simulink model "IntegratedpmsmmotorofEV"  (R2025b)
settings: Solver=VariableStepAuto  StartTime=0.0  StopTime=400  RelTol=1e-3
values from neighbouring files (symbols this model uses):
  av = 1 / 1.475    (= 0.677966101695)    [variable_initialization.m]
  ig = 9    [variable_initialization.m]
  Ld = 1e-4    (= 0.0001)    [variable_initialization.m]
  phi = 0.23    [variable_initialization.m]
  Reff = 0.3    [variable_initialization.m]
  Rs = 0.00475    [variable_initialization.m]
  Zp = 3    [variable_initialization.m]
libraries: slpidlib x2
settings Model: Creator=HS TRADER  LastModifiedBy=sheik
settings RTWCC: GPUComputeCapability=3.5

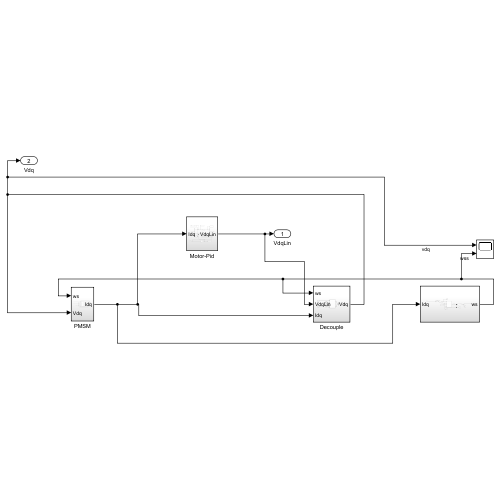
[thumbnail: Simulink's stored preview of the top-level diagram]
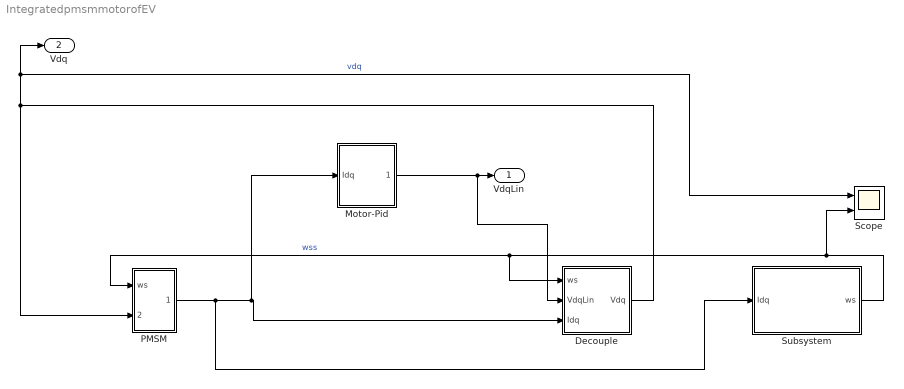
== system IntegratedpmsmmotorofEV ==
  Decouple : Subsystem
  Motor-Pid : Subsystem
  PMSM : Subsystem
  Scope : Scope  NumInputPorts=2
      settings: ActiveDisplayYMinimum=-1  ActiveDisplayYMaximum=1  DataLoggingVariableName=ScopeData2
  Subsystem : Subsystem
  VdqLin : Outport
  Vdq : Outport  Port=2
  wires:
  Motor-Pid/1(VdqLin) -> Decouple/2(VdqLin), VdqLin/1
  Decouple/1(Vdq) -> PMSM/2(Vdq), Scope/1, Vdq/1  "vdq"
  PMSM/1(Idq) -> Subsystem/1(Idq), Motor-Pid/1(Idq), Decouple/3(Idq)
  Subsystem/1(ws) -> Scope/2, Decouple/1(ws), PMSM/1(ws)  "wss"

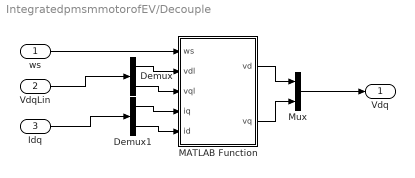
== system IntegratedpmsmmotorofEV/Decouple ==
  ws : Inport
  VdqLin : Inport  Port=2
  Idq : Inport  Port=3
  Demux : Demux  Outputs=2
  Demux1 : Demux  Outputs=2
  MATLAB Function : MATLAB Function  TreatAsAtomicUnit=on
  Mux : Mux  Inputs=2
  Vdq : Outport
  wires:
  Demux1/2 -> MATLAB Function/5(id)
  Demux/2 -> MATLAB Function/3(vql)
  Mux/1 -> Vdq/1
  Demux/1 -> MATLAB Function/2(vdl)
  MATLAB Function/1(vd) -> Mux/1
  VdqLin/1 -> Demux/1
  ws/1 -> MATLAB Function/1(ws)
  Demux1/1 -> MATLAB Function/4(iq)
  MATLAB Function/2(vq) -> Mux/2
  Idq/1 -> Demux1/1

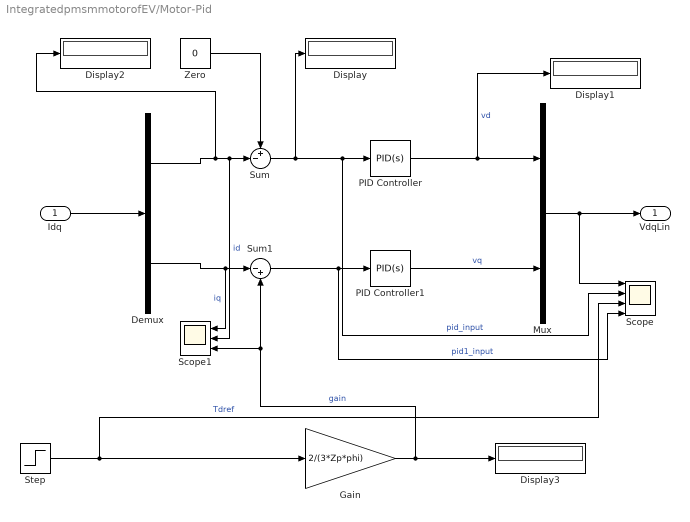
== system IntegratedpmsmmotorofEV/Motor-Pid ==
  Idq : Inport
  Demux : Demux  Outputs=2
  Display{,1..3} (4 alike) : Display
  Gain : Gain  Gain=2/(3*Zp*phi)
  Mux : Mux  Inputs=2
  PID Controller : slpidlib/PID Controller  Controller=PID  Form=Parallel  TimeDomain=Continuous-time  UseExternalTs=off  SampleTime=-1  IntegratorMethod=Forward Euler  FilterMethod=Forward Euler  ControllerParametersSource=internal  P=av  I=(Rs/Ld)*av  UseKiTs=off  D=0  UseExternalDerivativeSource=off  N=100  UseFilter=on  TunerSelectOption=Transfer Function Based (PID Tuner App)  InitialConditionSource=internal  InitialConditionForIntegrator=0  InitialConditionForFilter=0  DifferentiatorICPrevScaledInput=0  ExternalReset=none  TrackingMode=off  Kt=1  LimitOutput=off  SatLimitsSource=internal  UpperSaturationLimit=inf  LowerSaturationLimit=-inf  LinearizeAsGain=on  AntiWindupMode=none  Kb=1  LimitIntegrator=off  UpperIntegratorSaturationLimit=inf  LowerIntegratorSaturationLimit=-inf  POutMin=[]  POutMax=[]  IOutMin=[]  IOutMax=[]  DOutMin=[]  DOutMax=[]  NOutMin=[]  NOutMax=[]  SumOutMin=[]  SumOutMax=[]  SaturationOutMin=[]  SaturationOutMax=[]  PParamMin=[]  PParamMax=[]  IParamMin=[]  IParamMax=[]  DParamMin=[]  DParamMax=[]  NParamMin=[]  NParamMax=[]  KbParamMin=[]  KbParamMax=[]  KtParamMin=[]  KtParamMax=[]  KbOutMin=[]  KbOutMax=[]  KtOutMin=[]  KtOutMax=[]  IntegratorOutMin=[]  IntegratorOutMax=[]  FilterOutMin=[]  FilterOutMax=[]  SumI1OutMin=[]  SumI1OutMax=[]  SumI2OutMin=[]  SumI2OutMax=[]  SumI3OutMin=[]  SumI3OutMax=[]  SumI4OutMin=[]  SumI4OutMax=[]  SumDOutMin=[]  SumDOutMax=[]  DifferentiatorOutMin=[]  DifferentiatorOutMax=[]  FilterDiffOutCoefMin=[]  FilterDiffOutCoefMax=[]  ReciprocalOutMin=[]  ReciprocalOutMax=[]  SumDenOutMin=[]  SumDenOutMax=[]  SumNumOutMin=[]  SumNumOutMax=[]  DivideOutMin=[]  DivideOutMax=[]  UdiffTsProdOutMin=[]  UdiffTsProdOutMax=[]  NTsProdOutMin=[]  NTsProdOutMax=[]  UintegralTsProdOutMin=[]  UintegralTsProdOutMax=[]  UngainTsProdOutMin=[]  UngainTsProdOutMax=[]  ClampingZeroOutDataTypeStr=Inherit: Inherit via back propagation  ClampingZeroOutMin=[]  ClampingZeroOutMax=[]  FilterDenConstantOutDataTypeStr=Inherit: Inherit via back propagation  FilterDenConstantOutMin=[]  FilterDenConstantOutMax=[]  PCopyOutDataTypeStr=Inherit: Inherit via back propagation  PCopyOutMin=[]  PCopyOutMax=[]  NCopyOutDataTypeStr=Inherit: Inherit via back propagation  NCopyOutMin=[]  NCopyOutMax=[]  IntegratorContinuousStateAttributes=''  IntegratorStateMustResolveToSignalObject=off  IntegratorRTWStateStorageClass=Auto  FilterContinuousStateAttributes=''  FilterStateMustResolveToSignalObject=off  FilterRTWStateStorageClass=Auto  ParallelPVariant=InternalParameters  IdealPVariant=Disabled  IVariant=InternalParameters  DVariant=InternalParameters  IntegratorVariant=Continuous  SatVariant=Disabled  AWVariant=Passthrough  PCopyVariant=Disabled  TRVariant=Disabled  FdbkBlocksVariant=Forward  IdealPFdbkVariant=Disabled  SatFdbkVariant=Disabled  DerivativeFilterVariant=ContFilter  NVariant=InternalParameters  NCopyVariant=Disabled  FilterICVariant=InternalICsFilter  IntegratorICVariant=InternalICs  ExternalResetVariant=Disabled  TRSumVariant=Passthrough  SumFdbkVariant=Disabled  SumVariant=Sum_PID  TsampFilterVariant=InternalTs  TsampNgainVariant=Passthrough  TsampIntegralVariant=Disabled_SignalSpec  ExternalSaturationOutDataTypeStr=Inherit: Same as second input  DerivativeSourceVariant=ErrorSignal  PreIntVariant=InternalPreInt
  PID Controller1 : slpidlib/PID Controller  Controller=PID  Form=Parallel  TimeDomain=Continuous-time  UseExternalTs=off  SampleTime=-1  IntegratorMethod=Forward Euler  FilterMethod=Forward Euler  ControllerParametersSource=internal  P=av  I=(Rs/Ld)*av  UseKiTs=off  D=0  UseExternalDerivativeSource=off  N=100  UseFilter=on  TunerSelectOption=Transfer Function Based (PID Tuner App)  InitialConditionSource=internal  InitialConditionForIntegrator=0  InitialConditionForFilter=0  DifferentiatorICPrevScaledInput=0  ExternalReset=none  TrackingMode=off  Kt=1  LimitOutput=off  SatLimitsSource=internal  UpperSaturationLimit=inf  LowerSaturationLimit=-inf  LinearizeAsGain=on  AntiWindupMode=none  Kb=1  LimitIntegrator=off  UpperIntegratorSaturationLimit=inf  LowerIntegratorSaturationLimit=-inf  POutMin=[]  POutMax=[]  IOutMin=[]  IOutMax=[]  DOutMin=[]  DOutMax=[]  NOutMin=[]  NOutMax=[]  SumOutMin=[]  SumOutMax=[]  SaturationOutMin=[]  SaturationOutMax=[]  PParamMin=[]  PParamMax=[]  IParamMin=[]  IParamMax=[]  DParamMin=[]  DParamMax=[]  NParamMin=[]  NParamMax=[]  KbParamMin=[]  KbParamMax=[]  KtParamMin=[]  KtParamMax=[]  KbOutMin=[]  KbOutMax=[]  KtOutMin=[]  KtOutMax=[]  IntegratorOutMin=[]  IntegratorOutMax=[]  FilterOutMin=[]  FilterOutMax=[]  SumI1OutMin=[]  SumI1OutMax=[]  SumI2OutMin=[]  SumI2OutMax=[]  SumI3OutMin=[]  SumI3OutMax=[]  SumI4OutMin=[]  SumI4OutMax=[]  SumDOutMin=[]  SumDOutMax=[]  DifferentiatorOutMin=[]  DifferentiatorOutMax=[]  FilterDiffOutCoefMin=[]  FilterDiffOutCoefMax=[]  ReciprocalOutMin=[]  ReciprocalOutMax=[]  SumDenOutMin=[]  SumDenOutMax=[]  SumNumOutMin=[]  SumNumOutMax=[]  DivideOutMin=[]  DivideOutMax=[]  UdiffTsProdOutMin=[]  UdiffTsProdOutMax=[]  NTsProdOutMin=[]  NTsProdOutMax=[]  UintegralTsProdOutMin=[]  UintegralTsProdOutMax=[]  UngainTsProdOutMin=[]  UngainTsProdOutMax=[]  ClampingZeroOutDataTypeStr=Inherit: Inherit via back propagation  ClampingZeroOutMin=[]  ClampingZeroOutMax=[]  FilterDenConstantOutDataTypeStr=Inherit: Inherit via back propagation  FilterDenConstantOutMin=[]  FilterDenConstantOutMax=[]  PCopyOutDataTypeStr=Inherit: Inherit via back propagation  PCopyOutMin=[]  PCopyOutMax=[]  NCopyOutDataTypeStr=Inherit: Inherit via back propagation  NCopyOutMin=[]  NCopyOutMax=[]  IntegratorContinuousStateAttributes=''  IntegratorStateMustResolveToSignalObject=off  IntegratorRTWStateStorageClass=Auto  FilterContinuousStateAttributes=''  FilterStateMustResolveToSignalObject=off  FilterRTWStateStorageClass=Auto  ParallelPVariant=InternalParameters  IdealPVariant=Disabled  IVariant=InternalParameters  DVariant=InternalParameters  IntegratorVariant=Continuous  SatVariant=Disabled  AWVariant=Passthrough  PCopyVariant=Disabled  TRVariant=Disabled  FdbkBlocksVariant=Forward  IdealPFdbkVariant=Disabled  SatFdbkVariant=Disabled  DerivativeFilterVariant=ContFilter  NVariant=InternalParameters  NCopyVariant=Disabled  FilterICVariant=InternalICsFilter  IntegratorICVariant=InternalICs  ExternalResetVariant=Disabled  TRSumVariant=Passthrough  SumFdbkVariant=Disabled  SumVariant=Sum_PID  TsampFilterVariant=InternalTs  TsampNgainVariant=Passthrough  TsampIntegralVariant=Disabled_SignalSpec  ExternalSaturationOutDataTypeStr=Inherit: Same as second input  DerivativeSourceVariant=ErrorSignal  PreIntVariant=InternalPreInt
  Scope : Scope  NumInputPorts=4
      settings: ActiveDisplayYMinimum=-1  ActiveDisplayYMaximum=1
  Scope1 : Scope  NumInputPorts=3
      settings: ActiveDisplayYMinimum=-0.12860472493269859  ActiveDisplayYMaximum=1.0958441708195967
  Step : Step  SampleTime=0
  Sum : Sum  Inputs=+-|
  Sum1 : Sum  Inputs=|-+
  Zero : Constant  Value=0  OutDataTypeStr=Inherit: Inherit via back propagation
  VdqLin : Outport
  wires:
  Mux/1 -> VdqLin/1, Scope/1
  Sum/1 -> Display/1, Scope/2, PID Controller/1  "pid_input"
  Gain/1 -> Display3/1, Sum1/2, Scope1/3  "gain"
  PID Controller1/1 -> Mux/2  "vq"
  Demux/2 -> Scope1/1, Sum1/1  "iq"
  Demux/1 -> Display2/1, Scope1/2, Sum/2  "id"
  Step/1 -> Scope/3, Gain/1  "Tdref"
  Idq/1 -> Demux/1
  PID Controller/1 -> Display1/1, Mux/1  "vd"
  Sum1/1 -> Scope/4, PID Controller1/1  "pid1_input"
  Zero/1 -> Sum/1

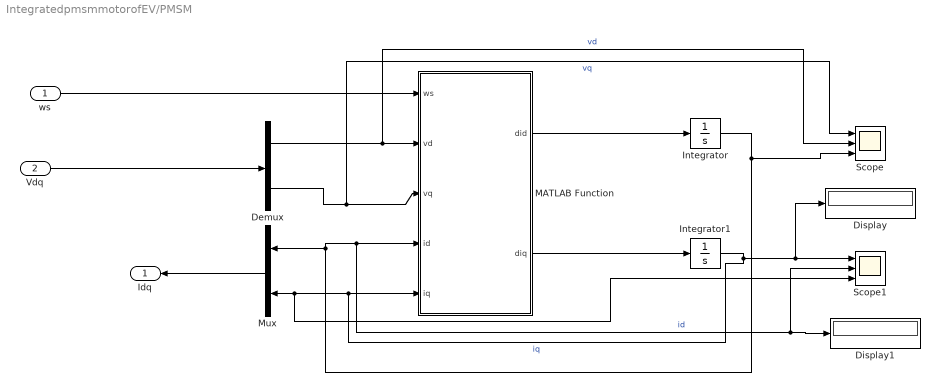
== system IntegratedpmsmmotorofEV/PMSM ==
  ws : Inport
  Vdq : Inport  Port=2
  Demux : Demux  Outputs=2
  Display : Display
  Display1 : Display
  Integrator : Integrator
  Integrator1 : Integrator
  MATLAB Function : MATLAB Function  TreatAsAtomicUnit=on
  Mux : Mux  Inputs=2
  Scope : Scope  NumInputPorts=3
      settings: ActiveDisplayYMinimum=-0.89375469680335762  ActiveDisplayYMaximum=0.89752600112387948
  Scope1 : Scope  NumInputPorts=3
      settings: ActiveDisplayYMinimum=-1  ActiveDisplayYMaximum=1
  Idq : Outport
  wires:
  Demux/2 -> Scope/1, MATLAB Function/3(vq)  "vq"
  ws/1 -> MATLAB Function/1(ws)
  Demux/1 -> Scope/2, MATLAB Function/2(vd)  "vd"
  Integrator1/1 -> Display/1, Scope1/1, MATLAB Function/5(iq), Scope1/3, Mux/2  "iq"
  MATLAB Function/2(diq) -> Integrator1/1
  MATLAB Function/1(did) -> Integrator/1
  Integrator/1 -> Scope/3, Display1/1, Scope1/2, MATLAB Function/4(id), Mux/1  "id"
  Mux/1 -> Idq/1
  Vdq/1 -> Demux/1

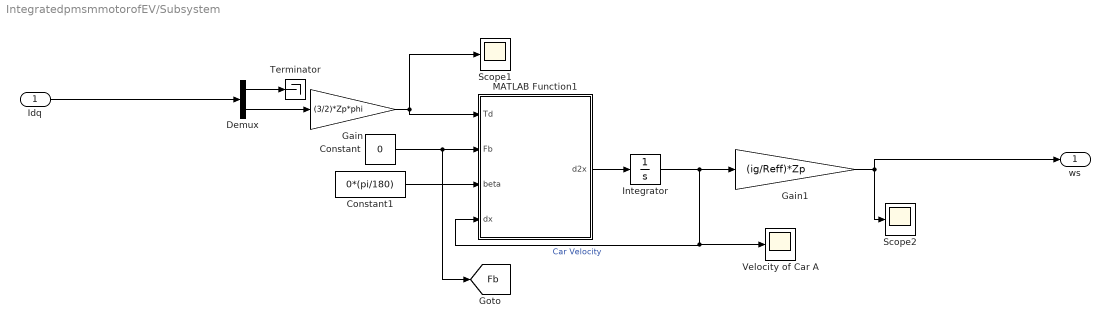
== system IntegratedpmsmmotorofEV/Subsystem ==
  Idq : Inport
  Constant : Constant  Value=0
  Constant1 : Constant  Value=0*(pi/180)
  Demux : Demux  Outputs=2
  Gain : Gain  Gain=(3/2)*Zp*phi
  Gain1 : Gain  Gain=(ig/Reff)*Zp
  Integrator : Integrator
  MATLAB Function1 : MATLAB Function  TreatAsAtomicUnit=on
  Scope1 : Scope
      settings: ActiveDisplayYMinimum=-60.1429  ActiveDisplayYMaximum=533.4162
  Scope2 : Scope
      settings: ActiveDisplayYMinimum=-759.67165918570618  ActiveDisplayYMaximum=6837.0447028710169  DataLoggingVariableName=ScopeData4
  Terminator : Terminator
  Velocity of Car A : Scope
      settings: ActiveDisplayYMinimum=-5.7063552940319857  ActiveDisplayYMaximum=51.357109308032818
  ws : Outport
  tag scope: Fb=global
  wires:
  Integrator/1 -> MATLAB Function1/4(dx), Velocity of Car A/1, Gain1/1  "Car Velocity"
  Demux/1 -> Terminator/1
  MATLAB Function1/1(d2x) -> Integrator/1
  Gain1/1 -> ws/1, Scope2/1
  Constant/1 -> [Fb], MATLAB Function1/2(Fb)
  Demux/2 -> Gain/1
  Gain/1 -> MATLAB Function1/1(Td), Scope1/1
  Constant1/1 -> MATLAB Function1/3(beta)
  Idq/1 -> Demux/1

== matlab function IntegratedpmsmmotorofEV/Decouple/MATLAB Function ==
  data: ws input; vd output; vdl input; vql input; iq input; id input; vq output
function [vd,vq]= decouple(ws,vdl,vql,iq,id)
Ld = 1e-4;
Lq = 1e-3;
phi = 0.23;
vd = -ws*Lq*iq + vdl*Ld;
vq = ws*phi + ws*Ld*id + vql*Lq;

== matlab function IntegratedpmsmmotorofEV/PMSM/MATLAB Function ==
  data: ws input; did output; vd input; vq input; id input; iq input; diq output
function [did,diq] = fcn(ws,vd,vq,id,iq)
Ld=1e-4;
Lq=1e-3;
Rs=0.00475;
phi=0.23;
did=ws*(Lq/Ld)*iq-(Rs/Ld)*id+(1/Ld)*vd;
diq=-ws*(1/Lq)*phi-ws*(Ld/Lq)*id-(Rs/Lq)*iq+(1/Lq)*vq;

== matlab function IntegratedpmsmmotorofEV/Subsystem/MATLAB Function1 ==
  data: Td input; d2x output; Fb input; beta input; dx input
function d2x = fcn(Td,Fb,beta,dx)
m=1992;
Reff=0.2413;
ig=9;
CR=0.0004;
CW=0.23;
g=9.81;
A=3.45;
Rho=1.1839;
Tw = ig*Td;
d2x = ((1/(m*Reff))*Tw)-CR*g*cos(beta)-((1/2)*CW*A*Rho*(dx.^2))/m-g*sin(beta)-(1/m)*Fb;
